simulink model "robust"  (R2022b)
settings: Solver=VariableStepAuto  StartTime=0.0  StopTime=25  RelTol=1e-3
values from neighbouring files (symbols this model uses):
  Beq = 2.0e-6    (= 2e-06)    [parameters.m]
  C = [1 0]    [parameters.m]
  degs2rpm = 60/360    (= 0.166666666667)    [parameters.m]
  Jeq = mot.J + mld.Jl / (gbox.N ^ 2)    [parameters.m]
  K1 = [K(1,2),K(1,3)]    [parameters.m]
  K2 = K(1,1)    [parameters.m]
  rads2rpm = 60/2/pi    (= 9.54929658551)    [parameters.m]
  Req = mot.R + Rs    [parameters.m]
  rpm2rads = 2*pi/60    (= 0.10471975512)    [parameters.m]
  sci = 1/sqrt(2)    [parameters.m]
  w_c = 2*pi*50    (= 314.159265359)    [parameters.m]
undefined symbols (not defined in the file or in its folder): drv, gbox, mld, mot
libraries: simulink x1
settings Model: Creator=nazanin  LastModifiedBy=nazanin
settings SolverCC: ZeroCrossAlgorithm=Adaptive
settings DebuggingCC: IgnoredZcDiagnostic=none

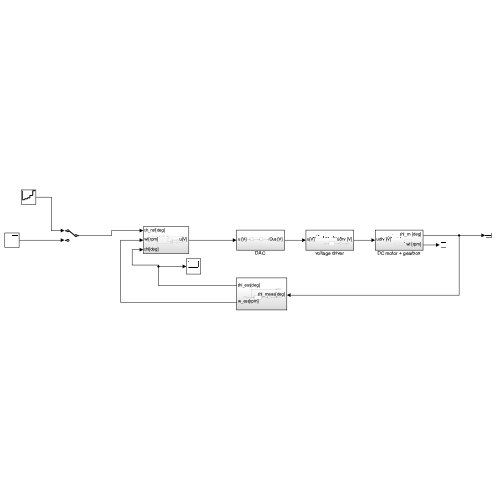
[thumbnail: Simulink's stored preview of the top-level diagram]
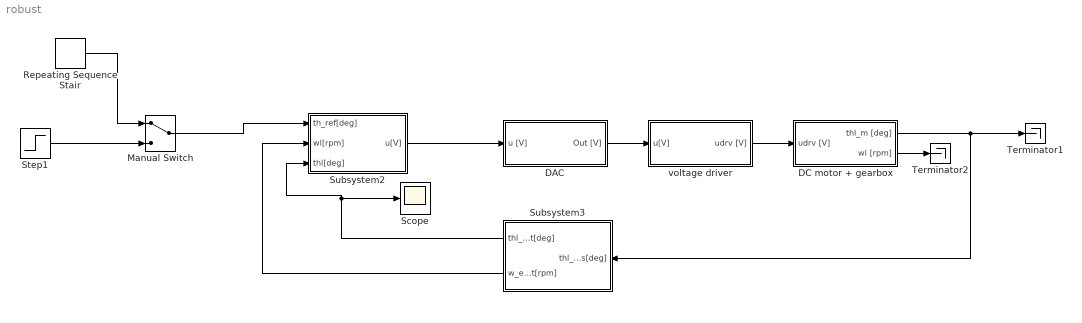
== system robust ==
  DAC : Subsystem
  DC motor + gearbox : Subsystem
  Manual Switch : ManualSwitch
  Repeating Sequence Stair : simulink/Sources/Repeating Sequence Stair  OutValues=[10 45 90 180 360].'  tsamp=5  OutMin=[]  OutMax=[]  OutDataTypeStr=double  OutputDataTypeScalingMode=double  OutDataType=fixdt(0,8)  ConRadixGroup=Best Precision: Vector-wise  OutScaling=2^-12
  Scope : Scope
  Step1 : Step  Time=0  After=70  SampleTime=0
  Subsystem2 : Subsystem
  Subsystem3 : Subsystem
  Terminator1 : Terminator
  Terminator2 : Terminator
  voltage driver : Subsystem
  wires:
  voltage driver/1(udrv [V]) -> DC motor + gearbox/1(udrv [V])
  DC motor + gearbox/2(wl [rpm]) -> Terminator2/1
  DAC/1(Out [V]) -> voltage driver/1(u[V])
  DC motor + gearbox/1(thl_m [deg]) -> Subsystem3/1(thl_meas[deg]), Terminator1/1
  Step1/1 -> Manual Switch/2
  Repeating Sequence Stair/1 -> Manual Switch/1
  Subsystem3/1(thl_est[deg]) -> Subsystem2/3(thl[deg]), Scope/1
  Subsystem3/2(w_est[rpm]) -> Subsystem2/2(wl[rpm])
  Manual Switch/1 -> Subsystem2/1(th_ref[deg])
  Subsystem2/1(u[V]) -> DAC/1(u [V])

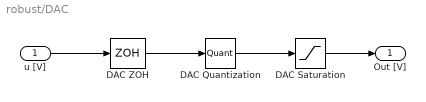
== system robust/DAC ==
  u [V] : Inport
  DAC Quantization : Quantizer  QuantizationInterval=20/(2^16 - 1)
  DAC Saturation : Saturate  UpperLimit=10  LowerLimit=-10
  DAC ZOH : ZeroOrderHold  SampleTime=0.001
  Out [V] : Outport
  wires:
  DAC Saturation/1 -> Out [V]/1
  DAC Quantization/1 -> DAC Saturation/1
  DAC ZOH/1 -> DAC Quantization/1
  u [V]/1 -> DAC ZOH/1

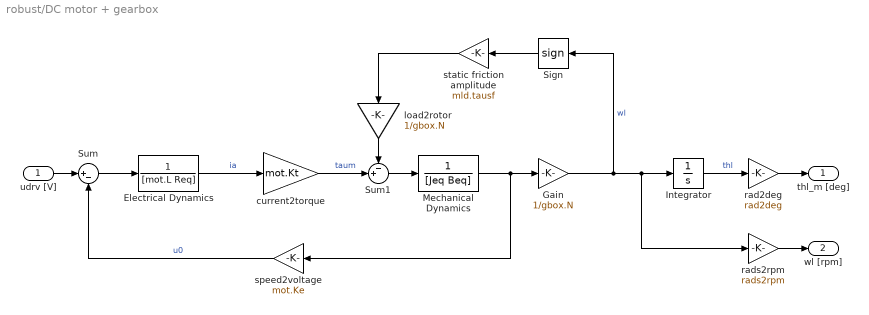
== system robust/DC motor + gearbox ==
  udrv [V] : Inport
  Electrical Dynamics : TransferFcn  Denominator=[mot.L Req]
  Gain : Gain  Gain=1/gbox.N
  Integrator : Integrator
  Mechanical Dynamics : TransferFcn  Denominator=[Jeq Beq]
  Sign : Signum  ZeroCross=off
  Sum : Sum  Inputs=|+-
  Sum1 : Sum  Inputs=-+|
  current2torque : Gain  Gain=mot.Kt
  load2rotor : Gain  Gain=1/gbox.N
  rad2deg : Gain  Gain=rad2deg
  rads2rpm : Gain  Gain=rads2rpm
  speed2voltage : Gain  Gain=mot.Ke
  static friction amplitude : Gain  Gain=mld.tausf
  thl_m [deg] : Outport
  wl [rpm] : Outport  Port=2
  wires:
  rads2rpm/1 -> wl [rpm]/1
  current2torque/1 -> Sum1/2  "taum"
  Mechanical Dynamics/1 -> Gain/1, speed2voltage/1
  Sign/1 -> static friction amplitude/1
  speed2voltage/1 -> Sum/2  "u0"
  Integrator/1 -> rad2deg/1  "thl"
  Sum/1 -> Electrical Dynamics/1
  rad2deg/1 -> thl_m [deg]/1
  udrv [V]/1 -> Sum/1
  Electrical Dynamics/1 -> current2torque/1  "ia"
  static friction amplitude/1 -> load2rotor/1
  Gain/1 -> rads2rpm/1, Integrator/1, Sign/1  "wl"
  Sum1/1 -> Mechanical Dynamics/1
  load2rotor/1 -> Sum1/1

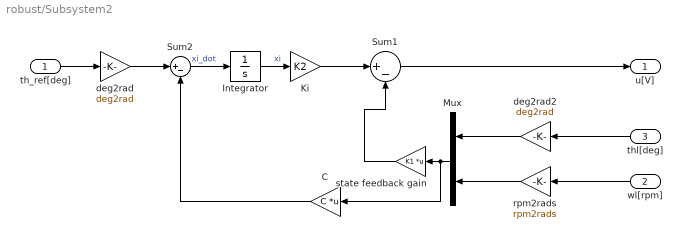
== system robust/Subsystem2 ==
  th_ref[deg] : Inport
  wl[rpm] : Inport  Port=2
  thl[deg] : Inport  Port=3
  C : Gain  Gain=C  Multiplication=Matrix(K*u)
  Integrator : Integrator
  Ki : Gain  Gain=K2
  Mux : Mux  Inputs=2
  Sum1 : Sum  Inputs=|+-
  Sum2 : Sum  Inputs=|+-
  deg2rad : Gain  Gain=deg2rad
  deg2rad2 : Gain  Gain=deg2rad
  rpm2rads : Gain  Gain=rpm2rads
  state feedback gain : Gain  Gain=K1  Multiplication=Matrix(K*u)
  u[V] : Outport
  wires:
  Sum1/1 -> u[V]/1
  thl[deg]/1 -> deg2rad2/1
  wl[rpm]/1 -> rpm2rads/1
  th_ref[deg]/1 -> deg2rad/1
  deg2rad2/1 -> Mux/1
  rpm2rads/1 -> Mux/2
  Mux/1 -> C/1, state feedback gain/1
  deg2rad/1 -> Sum2/1
  C/1 -> Sum2/2
  state feedback gain/1 -> Sum1/2
  Integrator/1 -> Ki/1  "xi"
  Sum2/1 -> Integrator/1  "xi_dot"
  Ki/1 -> Sum1/1

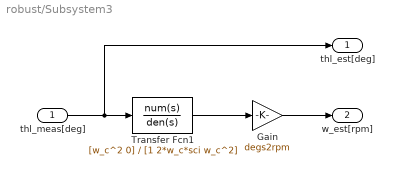
== system robust/Subsystem3 ==
  thl_meas[deg] : Inport
  Gain : Gain  Gain=degs2rpm
  Transfer Fcn1 : TransferFcn  Numerator=[w_c^2 0]  Denominator=[1 2*w_c*sci w_c^2]
  thl_est[deg] : Outport
  w_est[rpm] : Outport  Port=2
  wires:
  Gain/1 -> w_est[rpm]/1
  Transfer Fcn1/1 -> Gain/1
  thl_meas[deg]/1 -> Transfer Fcn1/1, thl_est[deg]/1

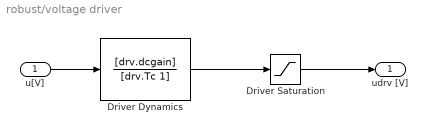
== system robust/voltage driver ==
  u[V] : Inport
  Driver Dynamics : TransferFcn  Numerator=[drv.dcgain]  Denominator=[drv.Tc 1]
  Driver Saturation : Saturate  UpperLimit=12  LowerLimit=-12
  udrv [V] : Outport
  wires:
  Driver Dynamics/1 -> Driver Saturation/1
  Driver Saturation/1 -> udrv [V]/1
  u[V]/1 -> Driver Dynamics/1
